simulink model "RADTRANS001"  (R2020b)
settings: Solver=VariableStepAuto  StartTime=0.0  StopTime=10.0  RelTol=1e-3
undefined symbols (not defined in the file): Line_110_C, Line_110_L, Line_110_R, Line_220_C, Line_220_L, Line_220_R, Line_35_C, Line_35_L, Line_35_R, Line_6_L, Line_6_R, Sys_f_Hz, Sys_V_net_kV, Tr_110_35_L_pu, Tr_110_35_R_pu, Tr_110_35_Sn_VA, Tr_110_35_V_HV_kV, Tr_110_35_V_LV_kV, Tr_110_6_L_pu, Tr_110_6_R_pu, Tr_110_6_Sn_VA, Tr_110_6_V_HV_kV, Tr_110_6_V_LV_kV, Tr_220_110_L_pu, Tr_220_110_R_pu, Tr_220_110_Sn_VA, Tr_220_110_V_HV_kV, Tr_220_110_V_LV_kV, Tr_35_04_L_pu, Tr_35_04_R_pu, Tr_35_04_Sn_VA, Tr_35_04_V_HV_kV, Tr_35_04_V_LV_kV, Tr_6_04_L_pu, Tr_6_04_R_pu, Tr_6_04_Sn_VA, Tr_6_04_V_HV_kV, Tr_6_04_V_LV_kV, Ts_powergui
libraries: dspstat3 x240, powerlib x169, powerlib_meascontrol x60
(part 4 of 6)

== system RADTRANS001/M_IN_Город_5_2 ==
  Iptg_55 : Display
      settings: Format=bank
  PQptg_55 : Scope  NumInputPorts=2
  "Power0 (3ph, Instantaneous)" : powerlib_meascontrol/Measurements/Power (3ph, Instantaneous)
  Pptg_55 : Display
      settings: Format=bank
  Qptg_55 : Display
      settings: Format=bank
  RMS3 : dspstat3/RMS  run=off  directionMode=Each column  dimension=1  InputProcessing=Columns as channels (frame based)  reset_popup=None
  RMS4 : dspstat3/RMS  run=off  directionMode=Each column  dimension=1  InputProcessing=Columns as channels (frame based)  reset_popup=None
  RMS55 : dspstat3/RMS  run=off  directionMode=Each column  dimension=1  InputProcessing=Columns as channels (frame based)  reset_popup=None
  RMSpt_55 : dspstat3/RMS  run=off  directionMode=Each column  dimension=1  InputProcessing=Columns as channels (frame based)  reset_popup=None
  Real-Ima to Complex : RealImagToComplex
  S : Abs
  SSptg_55 : Scope
  Sptg_55 : Display
      settings: Format=bank
  Three-Phase V-I Measurementpt_55 : powerlib/Measurements/Three-Phase V-I Measurement  VoltageMeasurement=phase-to-ground  SetLabelV=off  LabelV=Vabc  Vpu=off  VpuLL=off  CurrentMeasurement=yes  SetLabelI=off  LabelI=Iabc  Ipu=off  Pbase=100e6  Vbase=500e3  OutputType=Complex  PhasorSimulation=off  PSBequivalent=0
  UIptg_55 : Scope  NumInputPorts=2
  Uptg_55 : Display
      settings: Format=bank
  a : PMIOPort  Side=Right
  b : PMIOPort  Port=2  Side=Right
  c : PMIOPort  Port=3  Side=Right
  A : PMIOPort  Port=4  Side=Left
  B : PMIOPort  Port=5  Side=Left
  C : PMIOPort  Port=6  Side=Left
  tag scope: I_ptg_55=global, P_ptg_55=global, Q_ptg_55=global, S_ptg_55=global, U_ptg_55=global
  wires:
  S/1 -> [S_ptg_55]
  Real-Ima to Complex/1 -> S/1
  [S_ptg_55] -> Sptg_55/1
  [S_ptg_55] -> SSptg_55/1
  [P_ptg_55] -> RMSpt_55/1
  RMSpt_55/1 -> Pptg_55/1
  RMS55/1 -> Qptg_55/1
  [U_ptg_55] -> RMS3/1
  RMS3/1 -> Uptg_55/1
  [P_ptg_55] -> Real-Ima to Complex/1
  [Q_ptg_55] -> RMS55/1
  [I_ptg_55] -> RMS4/1
  RMS4/1 -> Iptg_55/1
  [U_ptg_55] -> UIptg_55/1  "U"
  [P_ptg_55] -> PQptg_55/1  "P"
  [I_ptg_55] -> UIptg_55/2  "I"
  Three-Phase V-I Measurementpt_55/1 -> [U_ptg_55]
  [Q_ptg_55] -> Real-Ima to Complex/2
  Three-Phase V-I Measurementpt_55/2 -> [I_ptg_55]
  [U_ptg_55] -> "Power0 (3ph, Instantaneous)"/1
  [I_ptg_55] -> "Power0 (3ph, Instantaneous)"/2
  "Power0 (3ph, Instantaneous)"/2 -> [Q_ptg_55]
  "Power0 (3ph, Instantaneous)"/1 -> [P_ptg_55]
  [Q_ptg_55] -> PQptg_55/2  "Q"
  connections:
  Three-Phase V-I Measurementpt_55/LConn1 -- A/RConn1
  Three-Phase V-I Measurementpt_55/RConn1 -- a/RConn1
  Three-Phase V-I Measurementpt_55/LConn2 -- B/RConn1
  Three-Phase V-I Measurementpt_55/LConn3 -- C/RConn1
  Three-Phase V-I Measurementpt_55/RConn3 -- c/RConn1
  Three-Phase V-I Measurementpt_55/RConn2 -- b/RConn1

== system RADTRANS001/M_IN_Город_5_3 ==
  Iptg_57 : Display
      settings: Format=bank
  PQptg_57 : Scope  NumInputPorts=2
  "Power0 (3ph, Instantaneous)" : powerlib_meascontrol/Measurements/Power (3ph, Instantaneous)
  Pptg_57 : Display
      settings: Format=bank
  Qptg_57 : Display
      settings: Format=bank
  RMS3 : dspstat3/RMS  run=off  directionMode=Each column  dimension=1  InputProcessing=Columns as channels (frame based)  reset_popup=None
  RMS4 : dspstat3/RMS  run=off  directionMode=Each column  dimension=1  InputProcessing=Columns as channels (frame based)  reset_popup=None
  RMS57 : dspstat3/RMS  run=off  directionMode=Each column  dimension=1  InputProcessing=Columns as channels (frame based)  reset_popup=None
  RMSpt_57 : dspstat3/RMS  run=off  directionMode=Each column  dimension=1  InputProcessing=Columns as channels (frame based)  reset_popup=None
  Real-Ima to Complex : RealImagToComplex
  S : Abs
  SSptg_57 : Scope
  Sptg_57 : Display
      settings: Format=bank
  Three-Phase V-I Measurementpt_57 : powerlib/Measurements/Three-Phase V-I Measurement  VoltageMeasurement=phase-to-ground  SetLabelV=off  LabelV=Vabc  Vpu=off  VpuLL=off  CurrentMeasurement=yes  SetLabelI=off  LabelI=Iabc  Ipu=off  Pbase=100e6  Vbase=500e3  OutputType=Complex  PhasorSimulation=off  PSBequivalent=0
  UIptg_57 : Scope  NumInputPorts=2
  Uptg_57 : Display
      settings: Format=bank
  a : PMIOPort  Side=Right
  b : PMIOPort  Port=2  Side=Right
  c : PMIOPort  Port=3  Side=Right
  A : PMIOPort  Port=4  Side=Left
  B : PMIOPort  Port=5  Side=Left
  C : PMIOPort  Port=6  Side=Left
  tag scope: I_ptg_57=global, P_ptg_57=global, Q_ptg_57=global, S_ptg_57=global, U_ptg_57=global
  wires:
  S/1 -> [S_ptg_57]
  Real-Ima to Complex/1 -> S/1
  [S_ptg_57] -> Sptg_57/1
  [S_ptg_57] -> SSptg_57/1
  [P_ptg_57] -> RMSpt_57/1
  RMSpt_57/1 -> Pptg_57/1
  RMS57/1 -> Qptg_57/1
  [U_ptg_57] -> RMS3/1
  RMS3/1 -> Uptg_57/1
  [P_ptg_57] -> Real-Ima to Complex/1
  [Q_ptg_57] -> RMS57/1
  [I_ptg_57] -> RMS4/1
  RMS4/1 -> Iptg_57/1
  [U_ptg_57] -> UIptg_57/1  "U"
  [P_ptg_57] -> PQptg_57/1  "P"
  [I_ptg_57] -> UIptg_57/2  "I"
  Three-Phase V-I Measurementpt_57/1 -> [U_ptg_57]
  [Q_ptg_57] -> Real-Ima to Complex/2
  Three-Phase V-I Measurementpt_57/2 -> [I_ptg_57]
  [U_ptg_57] -> "Power0 (3ph, Instantaneous)"/1
  [I_ptg_57] -> "Power0 (3ph, Instantaneous)"/2
  "Power0 (3ph, Instantaneous)"/2 -> [Q_ptg_57]
  "Power0 (3ph, Instantaneous)"/1 -> [P_ptg_57]
  [Q_ptg_57] -> PQptg_57/2  "Q"
  connections:
  Three-Phase V-I Measurementpt_57/LConn1 -- A/RConn1
  Three-Phase V-I Measurementpt_57/RConn1 -- a/RConn1
  Three-Phase V-I Measurementpt_57/LConn2 -- B/RConn1
  Three-Phase V-I Measurementpt_57/LConn3 -- C/RConn1
  Three-Phase V-I Measurementpt_57/RConn3 -- c/RConn1
  Three-Phase V-I Measurementpt_57/RConn2 -- b/RConn1

== system RADTRANS001/M_IN_Город_5_4 ==
  Iptg_59 : Display
      settings: Format=bank
  PQptg_59 : Scope  NumInputPorts=2
  "Power0 (3ph, Instantaneous)" : powerlib_meascontrol/Measurements/Power (3ph, Instantaneous)
  Pptg_59 : Display
      settings: Format=bank
  Qptg_59 : Display
      settings: Format=bank
  RMS3 : dspstat3/RMS  run=off  directionMode=Each column  dimension=1  InputProcessing=Columns as channels (frame based)  reset_popup=None
  RMS4 : dspstat3/RMS  run=off  directionMode=Each column  dimension=1  InputProcessing=Columns as channels (frame based)  reset_popup=None
  RMS59 : dspstat3/RMS  run=off  directionMode=Each column  dimension=1  InputProcessing=Columns as channels (frame based)  reset_popup=None
  RMSpt_59 : dspstat3/RMS  run=off  directionMode=Each column  dimension=1  InputProcessing=Columns as channels (frame based)  reset_popup=None
  Real-Ima to Complex : RealImagToComplex
  S : Abs
  SSptg_59 : Scope
  Sptg_59 : Display
      settings: Format=bank
  Three-Phase V-I Measurementpt_59 : powerlib/Measurements/Three-Phase V-I Measurement  VoltageMeasurement=phase-to-ground  SetLabelV=off  LabelV=Vabc  Vpu=off  VpuLL=off  CurrentMeasurement=yes  SetLabelI=off  LabelI=Iabc  Ipu=off  Pbase=100e6  Vbase=500e3  OutputType=Complex  PhasorSimulation=off  PSBequivalent=0
  UIptg_59 : Scope  NumInputPorts=2
  Uptg_59 : Display
      settings: Format=bank
  a : PMIOPort  Side=Right
  b : PMIOPort  Port=2  Side=Right
  c : PMIOPort  Port=3  Side=Right
  A : PMIOPort  Port=4  Side=Left
  B : PMIOPort  Port=5  Side=Left
  C : PMIOPort  Port=6  Side=Left
  tag scope: I_ptg_59=global, P_ptg_59=global, Q_ptg_59=global, S_ptg_59=global, U_ptg_59=global
  wires:
  S/1 -> [S_ptg_59]
  Real-Ima to Complex/1 -> S/1
  [S_ptg_59] -> Sptg_59/1
  [S_ptg_59] -> SSptg_59/1
  [P_ptg_59] -> RMSpt_59/1
  RMSpt_59/1 -> Pptg_59/1
  RMS59/1 -> Qptg_59/1
  [U_ptg_59] -> RMS3/1
  RMS3/1 -> Uptg_59/1
  [P_ptg_59] -> Real-Ima to Complex/1
  [Q_ptg_59] -> RMS59/1
  [I_ptg_59] -> RMS4/1
  RMS4/1 -> Iptg_59/1
  [U_ptg_59] -> UIptg_59/1  "U"
  [P_ptg_59] -> PQptg_59/1  "P"
  [I_ptg_59] -> UIptg_59/2  "I"
  Three-Phase V-I Measurementpt_59/1 -> [U_ptg_59]
  [Q_ptg_59] -> Real-Ima to Complex/2
  Three-Phase V-I Measurementpt_59/2 -> [I_ptg_59]
  [U_ptg_59] -> "Power0 (3ph, Instantaneous)"/1
  [I_ptg_59] -> "Power0 (3ph, Instantaneous)"/2
  "Power0 (3ph, Instantaneous)"/2 -> [Q_ptg_59]
  "Power0 (3ph, Instantaneous)"/1 -> [P_ptg_59]
  [Q_ptg_59] -> PQptg_59/2  "Q"
  connections:
  Three-Phase V-I Measurementpt_59/LConn1 -- A/RConn1
  Three-Phase V-I Measurementpt_59/RConn1 -- a/RConn1
  Three-Phase V-I Measurementpt_59/LConn2 -- B/RConn1
  Three-Phase V-I Measurementpt_59/LConn3 -- C/RConn1
  Three-Phase V-I Measurementpt_59/RConn3 -- c/RConn1
  Three-Phase V-I Measurementpt_59/RConn2 -- b/RConn1

== system RADTRANS001/M_IN_Завод_1_1 ==
  Iptg_1 : Display
      settings: Format=bank
  PQptg_1 : Scope  NumInputPorts=2
  "Power0 (3ph, Instantaneous)" : powerlib_meascontrol/Measurements/Power (3ph, Instantaneous)
  Pptg_1 : Display
      settings: Format=bank
  Qptg_1 : Display
      settings: Format=bank
  RMS1 : dspstat3/RMS  run=off  directionMode=Each column  dimension=1  InputProcessing=Columns as channels (frame based)  reset_popup=None
  RMS3 : dspstat3/RMS  run=off  directionMode=Each column  dimension=1  InputProcessing=Columns as channels (frame based)  reset_popup=None
  RMS4 : dspstat3/RMS  run=off  directionMode=Each column  dimension=1  InputProcessing=Columns as channels (frame based)  reset_popup=None
  RMSpt_1 : dspstat3/RMS  run=off  directionMode=Each column  dimension=1  InputProcessing=Columns as channels (frame based)  reset_popup=None
  Real-Ima to Complex : RealImagToComplex
  S : Abs
  SSptg_1 : Scope
  Sptg_1 : Display
      settings: Format=bank
  Three-Phase V-I Measurementpt_1 : powerlib/Measurements/Three-Phase V-I Measurement  VoltageMeasurement=phase-to-ground  SetLabelV=off  LabelV=Vabc  Vpu=off  VpuLL=off  CurrentMeasurement=yes  SetLabelI=off  LabelI=Iabc  Ipu=off  Pbase=100e6  Vbase=500e3  OutputType=Complex  PhasorSimulation=off  PSBequivalent=0
  UIptg_1 : Scope  NumInputPorts=2
  Uptg_1 : Display
      settings: Format=bank
  a : PMIOPort  Side=Right
  b : PMIOPort  Port=2  Side=Right
  c : PMIOPort  Port=3  Side=Right
  A : PMIOPort  Port=4  Side=Left
  B : PMIOPort  Port=5  Side=Left
  C : PMIOPort  Port=6  Side=Left
  tag scope: I_ptg_1=global, P_ptg_1=global, Q_ptg_1=global, S_ptg_1=global, U_ptg_1=global
  wires:
  S/1 -> [S_ptg_1]
  Real-Ima to Complex/1 -> S/1
  [S_ptg_1] -> Sptg_1/1
  [S_ptg_1] -> SSptg_1/1
  [P_ptg_1] -> RMSpt_1/1
  RMSpt_1/1 -> Pptg_1/1
  RMS1/1 -> Qptg_1/1
  [U_ptg_1] -> RMS3/1
  RMS3/1 -> Uptg_1/1
  [P_ptg_1] -> Real-Ima to Complex/1
  [Q_ptg_1] -> RMS1/1
  [I_ptg_1] -> RMS4/1
  RMS4/1 -> Iptg_1/1
  [U_ptg_1] -> UIptg_1/1  "U"
  [P_ptg_1] -> PQptg_1/1  "P"
  [I_ptg_1] -> UIptg_1/2  "I"
  Three-Phase V-I Measurementpt_1/1 -> [U_ptg_1]
  [Q_ptg_1] -> Real-Ima to Complex/2
  Three-Phase V-I Measurementpt_1/2 -> [I_ptg_1]
  [U_ptg_1] -> "Power0 (3ph, Instantaneous)"/1
  [I_ptg_1] -> "Power0 (3ph, Instantaneous)"/2
  "Power0 (3ph, Instantaneous)"/2 -> [Q_ptg_1]
  "Power0 (3ph, Instantaneous)"/1 -> [P_ptg_1]
  [Q_ptg_1] -> PQptg_1/2  "Q"
  connections:
  Three-Phase V-I Measurementpt_1/LConn1 -- A/RConn1
  Three-Phase V-I Measurementpt_1/RConn1 -- a/RConn1
  Three-Phase V-I Measurementpt_1/LConn2 -- B/RConn1
  Three-Phase V-I Measurementpt_1/LConn3 -- C/RConn1
  Three-Phase V-I Measurementpt_1/RConn3 -- c/RConn1
  Three-Phase V-I Measurementpt_1/RConn2 -- b/RConn1

== system RADTRANS001/M_IN_Завод_1_2 ==
  Iptg_3 : Display
      settings: Format=bank
  PQptg_3 : Scope  NumInputPorts=2
  "Power0 (3ph, Instantaneous)" : powerlib_meascontrol/Measurements/Power (3ph, Instantaneous)
  Pptg_3 : Display
      settings: Format=bank
  Qptg_3 : Display
      settings: Format=bank
  RMS0 : dspstat3/RMS  run=off  directionMode=Each column  dimension=1  InputProcessing=Columns as channels (frame based)  reset_popup=None
  RMS3 : dspstat3/RMS  run=off  directionMode=Each column  dimension=1  InputProcessing=Columns as channels (frame based)  reset_popup=None
  RMS4 : dspstat3/RMS  run=off  directionMode=Each column  dimension=1  InputProcessing=Columns as channels (frame based)  reset_popup=None
  RMSpt_3 : dspstat3/RMS  run=off  directionMode=Each column  dimension=1  InputProcessing=Columns as channels (frame based)  reset_popup=None
  Real-Ima to Complex : RealImagToComplex
  S : Abs
  SSptg_3 : Scope
  Sptg_3 : Display
      settings: Format=bank
  Three-Phase V-I Measurementpt_3 : powerlib/Measurements/Three-Phase V-I Measurement  VoltageMeasurement=phase-to-ground  SetLabelV=off  LabelV=Vabc  Vpu=off  VpuLL=off  CurrentMeasurement=yes  SetLabelI=off  LabelI=Iabc  Ipu=off  Pbase=100e6  Vbase=500e3  OutputType=Complex  PhasorSimulation=off  PSBequivalent=0
  UIptg_3 : Scope  NumInputPorts=2
  Uptg_3 : Display
      settings: Format=bank
  a : PMIOPort  Side=Right
  b : PMIOPort  Port=2  Side=Right
  c : PMIOPort  Port=3  Side=Right
  A : PMIOPort  Port=4  Side=Left
  B : PMIOPort  Port=5  Side=Left
  C : PMIOPort  Port=6  Side=Left
  tag scope: I_ptg_3=global, P_ptg_3=global, Q_ptg_3=global, S_ptg_3=global, U_ptg_3=global
  wires:
  S/1 -> [S_ptg_3]
  Real-Ima to Complex/1 -> S/1
  [S_ptg_3] -> Sptg_3/1
  [S_ptg_3] -> SSptg_3/1
  [P_ptg_3] -> RMSpt_3/1
  RMSpt_3/1 -> Pptg_3/1
  RMS0/1 -> Qptg_3/1
  [U_ptg_3] -> RMS3/1
  RMS3/1 -> Uptg_3/1
  [P_ptg_3] -> Real-Ima to Complex/1
  [Q_ptg_3] -> RMS0/1
  [I_ptg_3] -> RMS4/1
  RMS4/1 -> Iptg_3/1
  [U_ptg_3] -> UIptg_3/1  "U"
  [P_ptg_3] -> PQptg_3/1  "P"
  [I_ptg_3] -> UIptg_3/2  "I"
  Three-Phase V-I Measurementpt_3/1 -> [U_ptg_3]
  [Q_ptg_3] -> Real-Ima to Complex/2
  Three-Phase V-I Measurementpt_3/2 -> [I_ptg_3]
  [U_ptg_3] -> "Power0 (3ph, Instantaneous)"/1
  [I_ptg_3] -> "Power0 (3ph, Instantaneous)"/2
  "Power0 (3ph, Instantaneous)"/2 -> [Q_ptg_3]
  "Power0 (3ph, Instantaneous)"/1 -> [P_ptg_3]
  [Q_ptg_3] -> PQptg_3/2  "Q"
  connections:
  Three-Phase V-I Measurementpt_3/LConn1 -- A/RConn1
  Three-Phase V-I Measurementpt_3/RConn1 -- a/RConn1
  Three-Phase V-I Measurementpt_3/LConn2 -- B/RConn1
  Three-Phase V-I Measurementpt_3/LConn3 -- C/RConn1
  Three-Phase V-I Measurementpt_3/RConn3 -- c/RConn1
  Three-Phase V-I Measurementpt_3/RConn2 -- b/RConn1

== system RADTRANS001/M_IN_Завод_2_1 ==
  Iptg_13 : Display
      settings: Format=bank
  PQptg_13 : Scope  NumInputPorts=2
  "Power0 (3ph, Instantaneous)" : powerlib_meascontrol/Measurements/Power (3ph, Instantaneous)
  Pptg_13 : Display
      settings: Format=bank
  Qptg_13 : Display
      settings: Format=bank
  RMS13 : dspstat3/RMS  run=off  directionMode=Each column  dimension=1  InputProcessing=Columns as channels (frame based)  reset_popup=None
  RMS3 : dspstat3/RMS  run=off  directionMode=Each column  dimension=1  InputProcessing=Columns as channels (frame based)  reset_popup=None
  RMS4 : dspstat3/RMS  run=off  directionMode=Each column  dimension=1  InputProcessing=Columns as channels (frame based)  reset_popup=None
  RMSpt_13 : dspstat3/RMS  run=off  directionMode=Each column  dimension=1  InputProcessing=Columns as channels (frame based)  reset_popup=None
  Real-Ima to Complex : RealImagToComplex
  S : Abs
  SSptg_13 : Scope
  Sptg_13 : Display
      settings: Format=bank
  Three-Phase V-I Measurementpt_13 : powerlib/Measurements/Three-Phase V-I Measurement  VoltageMeasurement=phase-to-ground  SetLabelV=off  LabelV=Vabc  Vpu=off  VpuLL=off  CurrentMeasurement=yes  SetLabelI=off  LabelI=Iabc  Ipu=off  Pbase=100e6  Vbase=500e3  OutputType=Complex  PhasorSimulation=off  PSBequivalent=0
  UIptg_13 : Scope  NumInputPorts=2
  Uptg_13 : Display
      settings: Format=bank
  a : PMIOPort  Side=Right
  b : PMIOPort  Port=2  Side=Right
  c : PMIOPort  Port=3  Side=Right
  A : PMIOPort  Port=4  Side=Left
  B : PMIOPort  Port=5  Side=Left
  C : PMIOPort  Port=6  Side=Left
  tag scope: I_ptg_13=global, P_ptg_13=global, Q_ptg_13=global, S_ptg_13=global, U_ptg_13=global
  wires:
  S/1 -> [S_ptg_13]
  Real-Ima to Complex/1 -> S/1
  [S_ptg_13] -> Sptg_13/1
  [S_ptg_13] -> SSptg_13/1
  [P_ptg_13] -> RMSpt_13/1
  RMSpt_13/1 -> Pptg_13/1
  RMS13/1 -> Qptg_13/1
  [U_ptg_13] -> RMS3/1
  RMS3/1 -> Uptg_13/1
  [P_ptg_13] -> Real-Ima to Complex/1
  [Q_ptg_13] -> RMS13/1
  [I_ptg_13] -> RMS4/1
  RMS4/1 -> Iptg_13/1
  [U_ptg_13] -> UIptg_13/1  "U"
  [P_ptg_13] -> PQptg_13/1  "P"
  [I_ptg_13] -> UIptg_13/2  "I"
  Three-Phase V-I Measurementpt_13/1 -> [U_ptg_13]
  [Q_ptg_13] -> Real-Ima to Complex/2
  Three-Phase V-I Measurementpt_13/2 -> [I_ptg_13]
  [U_ptg_13] -> "Power0 (3ph, Instantaneous)"/1
  [I_ptg_13] -> "Power0 (3ph, Instantaneous)"/2
  "Power0 (3ph, Instantaneous)"/2 -> [Q_ptg_13]
  "Power0 (3ph, Instantaneous)"/1 -> [P_ptg_13]
  [Q_ptg_13] -> PQptg_13/2  "Q"
  connections:
  Three-Phase V-I Measurementpt_13/LConn1 -- A/RConn1
  Three-Phase V-I Measurementpt_13/RConn1 -- a/RConn1
  Three-Phase V-I Measurementpt_13/LConn2 -- B/RConn1
  Three-Phase V-I Measurementpt_13/LConn3 -- C/RConn1
  Three-Phase V-I Measurementpt_13/RConn3 -- c/RConn1
  Three-Phase V-I Measurementpt_13/RConn2 -- b/RConn1

== system RADTRANS001/M_IN_Завод_2_2 ==
  Iptg_15 : Display
      settings: Format=bank
  PQptg_15 : Scope  NumInputPorts=2
  "Power0 (3ph, Instantaneous)" : powerlib_meascontrol/Measurements/Power (3ph, Instantaneous)
  Pptg_15 : Display
      settings: Format=bank
  Qptg_15 : Display
      settings: Format=bank
  RMS15 : dspstat3/RMS  run=off  directionMode=Each column  dimension=1  InputProcessing=Columns as channels (frame based)  reset_popup=None
  RMS3 : dspstat3/RMS  run=off  directionMode=Each column  dimension=1  InputProcessing=Columns as channels (frame based)  reset_popup=None
  RMS4 : dspstat3/RMS  run=off  directionMode=Each column  dimension=1  InputProcessing=Columns as channels (frame based)  reset_popup=None
  RMSpt_15 : dspstat3/RMS  run=off  directionMode=Each column  dimension=1  InputProcessing=Columns as channels (frame based)  reset_popup=None
  Real-Ima to Complex : RealImagToComplex
  S : Abs
  SSptg_15 : Scope
  Sptg_15 : Display
      settings: Format=bank
  Three-Phase V-I Measurementpt_15 : powerlib/Measurements/Three-Phase V-I Measurement  VoltageMeasurement=phase-to-ground  SetLabelV=off  LabelV=Vabc  Vpu=off  VpuLL=off  CurrentMeasurement=yes  SetLabelI=off  LabelI=Iabc  Ipu=off  Pbase=100e6  Vbase=500e3  OutputType=Complex  PhasorSimulation=off  PSBequivalent=0
  UIptg_15 : Scope  NumInputPorts=2
  Uptg_15 : Display
      settings: Format=bank
  a : PMIOPort  Side=Right
  b : PMIOPort  Port=2  Side=Right
  c : PMIOPort  Port=3  Side=Right
  A : PMIOPort  Port=4  Side=Left
  B : PMIOPort  Port=5  Side=Left
  C : PMIOPort  Port=6  Side=Left
  tag scope: I_ptg_15=global, P_ptg_15=global, Q_ptg_15=global, S_ptg_15=global, U_ptg_15=global
  wires:
  S/1 -> [S_ptg_15]
  Real-Ima to Complex/1 -> S/1
  [S_ptg_15] -> Sptg_15/1
  [S_ptg_15] -> SSptg_15/1
  [P_ptg_15] -> RMSpt_15/1
  RMSpt_15/1 -> Pptg_15/1
  RMS15/1 -> Qptg_15/1
  [U_ptg_15] -> RMS3/1
  RMS3/1 -> Uptg_15/1
  [P_ptg_15] -> Real-Ima to Complex/1
  [Q_ptg_15] -> RMS15/1
  [I_ptg_15] -> RMS4/1
  RMS4/1 -> Iptg_15/1
  [U_ptg_15] -> UIptg_15/1  "U"
  [P_ptg_15] -> PQptg_15/1  "P"
  [I_ptg_15] -> UIptg_15/2  "I"
  Three-Phase V-I Measurementpt_15/1 -> [U_ptg_15]
  [Q_ptg_15] -> Real-Ima to Complex/2
  Three-Phase V-I Measurementpt_15/2 -> [I_ptg_15]
  [U_ptg_15] -> "Power0 (3ph, Instantaneous)"/1
  [I_ptg_15] -> "Power0 (3ph, Instantaneous)"/2
  "Power0 (3ph, Instantaneous)"/2 -> [Q_ptg_15]
  "Power0 (3ph, Instantaneous)"/1 -> [P_ptg_15]
  [Q_ptg_15] -> PQptg_15/2  "Q"
  connections:
  Three-Phase V-I Measurementpt_15/LConn1 -- A/RConn1
  Three-Phase V-I Measurementpt_15/RConn1 -- a/RConn1
  Three-Phase V-I Measurementpt_15/LConn2 -- B/RConn1
  Three-Phase V-I Measurementpt_15/LConn3 -- C/RConn1
  Three-Phase V-I Measurementpt_15/RConn3 -- c/RConn1
  Three-Phase V-I Measurementpt_15/RConn2 -- b/RConn1

== system RADTRANS001/M_IN_Завод_3_1 ==
  Iptg_25 : Display
      settings: Format=bank
  PQptg_25 : Scope  NumInputPorts=2
  "Power0 (3ph, Instantaneous)" : powerlib_meascontrol/Measurements/Power (3ph, Instantaneous)
  Pptg_25 : Display
      settings: Format=bank
  Qptg_25 : Display
      settings: Format=bank
  RMS25 : dspstat3/RMS  run=off  directionMode=Each column  dimension=1  InputProcessing=Columns as channels (frame based)  reset_popup=None
  RMS3 : dspstat3/RMS  run=off  directionMode=Each column  dimension=1  InputProcessing=Columns as channels (frame based)  reset_popup=None
  RMS4 : dspstat3/RMS  run=off  directionMode=Each column  dimension=1  InputProcessing=Columns as channels (frame based)  reset_popup=None
  RMSpt_25 : dspstat3/RMS  run=off  directionMode=Each column  dimension=1  InputProcessing=Columns as channels (frame based)  reset_popup=None
  Real-Ima to Complex : RealImagToComplex
  S : Abs
  SSptg_25 : Scope
  Sptg_25 : Display
      settings: Format=bank
  Three-Phase V-I Measurementpt_25 : powerlib/Measurements/Three-Phase V-I Measurement  VoltageMeasurement=phase-to-ground  SetLabelV=off  LabelV=Vabc  Vpu=off  VpuLL=off  CurrentMeasurement=yes  SetLabelI=off  LabelI=Iabc  Ipu=off  Pbase=100e6  Vbase=500e3  OutputType=Complex  PhasorSimulation=off  PSBequivalent=0
  UIptg_25 : Scope  NumInputPorts=2
  Uptg_25 : Display
      settings: Format=bank
  a : PMIOPort  Side=Right
  b : PMIOPort  Port=2  Side=Right
  c : PMIOPort  Port=3  Side=Right
  A : PMIOPort  Port=4  Side=Left
  B : PMIOPort  Port=5  Side=Left
  C : PMIOPort  Port=6  Side=Left
  tag scope: I_ptg_25=global, P_ptg_25=global, Q_ptg_25=global, S_ptg_25=global, U_ptg_25=global
  wires:
  S/1 -> [S_ptg_25]
  Real-Ima to Complex/1 -> S/1
  [S_ptg_25] -> Sptg_25/1
  [S_ptg_25] -> SSptg_25/1
  [P_ptg_25] -> RMSpt_25/1
  RMSpt_25/1 -> Pptg_25/1
  RMS25/1 -> Qptg_25/1
  [U_ptg_25] -> RMS3/1
  RMS3/1 -> Uptg_25/1
  [P_ptg_25] -> Real-Ima to Complex/1
  [Q_ptg_25] -> RMS25/1
  [I_ptg_25] -> RMS4/1
  RMS4/1 -> Iptg_25/1
  [U_ptg_25] -> UIptg_25/1  "U"
  [P_ptg_25] -> PQptg_25/1  "P"
  [I_ptg_25] -> UIptg_25/2  "I"
  Three-Phase V-I Measurementpt_25/1 -> [U_ptg_25]
  [Q_ptg_25] -> Real-Ima to Complex/2
  Three-Phase V-I Measurementpt_25/2 -> [I_ptg_25]
  [U_ptg_25] -> "Power0 (3ph, Instantaneous)"/1
  [I_ptg_25] -> "Power0 (3ph, Instantaneous)"/2
  "Power0 (3ph, Instantaneous)"/2 -> [Q_ptg_25]
  "Power0 (3ph, Instantaneous)"/1 -> [P_ptg_25]
  [Q_ptg_25] -> PQptg_25/2  "Q"
  connections:
  Three-Phase V-I Measurementpt_25/LConn1 -- A/RConn1
  Three-Phase V-I Measurementpt_25/RConn1 -- a/RConn1
  Three-Phase V-I Measurementpt_25/LConn2 -- B/RConn1
  Three-Phase V-I Measurementpt_25/LConn3 -- C/RConn1
  Three-Phase V-I Measurementpt_25/RConn3 -- c/RConn1
  Three-Phase V-I Measurementpt_25/RConn2 -- b/RConn1

== system RADTRANS001/M_IN_Завод_3_2 ==
  Iptg_27 : Display
      settings: Format=bank
  PQptg_27 : Scope  NumInputPorts=2
  "Power0 (3ph, Instantaneous)" : powerlib_meascontrol/Measurements/Power (3ph, Instantaneous)
  Pptg_27 : Display
      settings: Format=bank
  Qptg_27 : Display
      settings: Format=bank
  RMS27 : dspstat3/RMS  run=off  directionMode=Each column  dimension=1  InputProcessing=Columns as channels (frame based)  reset_popup=None
  RMS3 : dspstat3/RMS  run=off  directionMode=Each column  dimension=1  InputProcessing=Columns as channels (frame based)  reset_popup=None
  RMS4 : dspstat3/RMS  run=off  directionMode=Each column  dimension=1  InputProcessing=Columns as channels (frame based)  reset_popup=None
  RMSpt_27 : dspstat3/RMS  run=off  directionMode=Each column  dimension=1  InputProcessing=Columns as channels (frame based)  reset_popup=None
  Real-Ima to Complex : RealImagToComplex
  S : Abs
  SSptg_27 : Scope
  Sptg_27 : Display
      settings: Format=bank
  Three-Phase V-I Measurementpt_27 : powerlib/Measurements/Three-Phase V-I Measurement  VoltageMeasurement=phase-to-ground  SetLabelV=off  LabelV=Vabc  Vpu=off  VpuLL=off  CurrentMeasurement=yes  SetLabelI=off  LabelI=Iabc  Ipu=off  Pbase=100e6  Vbase=500e3  OutputType=Complex  PhasorSimulation=off  PSBequivalent=0
  UIptg_27 : Scope  NumInputPorts=2
  Uptg_27 : Display
      settings: Format=bank
  a : PMIOPort  Side=Right
  b : PMIOPort  Port=2  Side=Right
  c : PMIOPort  Port=3  Side=Right
  A : PMIOPort  Port=4  Side=Left
  B : PMIOPort  Port=5  Side=Left
  C : PMIOPort  Port=6  Side=Left
  tag scope: I_ptg_27=global, P_ptg_27=global, Q_ptg_27=global, S_ptg_27=global, U_ptg_27=global
  wires:
  S/1 -> [S_ptg_27]
  Real-Ima to Complex/1 -> S/1
  [S_ptg_27] -> Sptg_27/1
  [S_ptg_27] -> SSptg_27/1
  [P_ptg_27] -> RMSpt_27/1
  RMSpt_27/1 -> Pptg_27/1
  RMS27/1 -> Qptg_27/1
  [U_ptg_27] -> RMS3/1
  RMS3/1 -> Uptg_27/1
  [P_ptg_27] -> Real-Ima to Complex/1
  [Q_ptg_27] -> RMS27/1
  [I_ptg_27] -> RMS4/1
  RMS4/1 -> Iptg_27/1
  [U_ptg_27] -> UIptg_27/1  "U"
  [P_ptg_27] -> PQptg_27/1  "P"
  [I_ptg_27] -> UIptg_27/2  "I"
  Three-Phase V-I Measurementpt_27/1 -> [U_ptg_27]
  [Q_ptg_27] -> Real-Ima to Complex/2
  Three-Phase V-I Measurementpt_27/2 -> [I_ptg_27]
  [U_ptg_27] -> "Power0 (3ph, Instantaneous)"/1
  [I_ptg_27] -> "Power0 (3ph, Instantaneous)"/2
  "Power0 (3ph, Instantaneous)"/2 -> [Q_ptg_27]
  "Power0 (3ph, Instantaneous)"/1 -> [P_ptg_27]
  [Q_ptg_27] -> PQptg_27/2  "Q"
  connections:
  Three-Phase V-I Measurementpt_27/LConn1 -- A/RConn1
  Three-Phase V-I Measurementpt_27/RConn1 -- a/RConn1
  Three-Phase V-I Measurementpt_27/LConn2 -- B/RConn1
  Three-Phase V-I Measurementpt_27/LConn3 -- C/RConn1
  Three-Phase V-I Measurementpt_27/RConn3 -- c/RConn1
  Three-Phase V-I Measurementpt_27/RConn2 -- b/RConn1

== system RADTRANS001/M_IN_Завод_4_1 ==
  Iptg_37 : Display
      settings: Format=bank
  PQptg_37 : Scope  NumInputPorts=2
  "Power0 (3ph, Instantaneous)" : powerlib_meascontrol/Measurements/Power (3ph, Instantaneous)
  Pptg_37 : Display
      settings: Format=bank
  Qptg_37 : Display
      settings: Format=bank
  RMS3 : dspstat3/RMS  run=off  directionMode=Each column  dimension=1  InputProcessing=Columns as channels (frame based)  reset_popup=None
  RMS37 : dspstat3/RMS  run=off  directionMode=Each column  dimension=1  InputProcessing=Columns as channels (frame based)  reset_popup=None
  RMS4 : dspstat3/RMS  run=off  directionMode=Each column  dimension=1  InputProcessing=Columns as channels (frame based)  reset_popup=None
  RMSpt_37 : dspstat3/RMS  run=off  directionMode=Each column  dimension=1  InputProcessing=Columns as channels (frame based)  reset_popup=None
  Real-Ima to Complex : RealImagToComplex
  S : Abs
  SSptg_37 : Scope
  Sptg_37 : Display
      settings: Format=bank
  Three-Phase V-I Measurementpt_37 : powerlib/Measurements/Three-Phase V-I Measurement  VoltageMeasurement=phase-to-ground  SetLabelV=off  LabelV=Vabc  Vpu=off  VpuLL=off  CurrentMeasurement=yes  SetLabelI=off  LabelI=Iabc  Ipu=off  Pbase=100e6  Vbase=500e3  OutputType=Complex  PhasorSimulation=off  PSBequivalent=0
  UIptg_37 : Scope  NumInputPorts=2
  Uptg_37 : Display
      settings: Format=bank
  a : PMIOPort  Side=Right
  b : PMIOPort  Port=2  Side=Right
  c : PMIOPort  Port=3  Side=Right
  A : PMIOPort  Port=4  Side=Left
  B : PMIOPort  Port=5  Side=Left
  C : PMIOPort  Port=6  Side=Left
  tag scope: I_ptg_37=global, P_ptg_37=global, Q_ptg_37=global, S_ptg_37=global, U_ptg_37=global
  wires:
  S/1 -> [S_ptg_37]
  Real-Ima to Complex/1 -> S/1
  [S_ptg_37] -> Sptg_37/1
  [S_ptg_37] -> SSptg_37/1
  [P_ptg_37] -> RMSpt_37/1
  RMSpt_37/1 -> Pptg_37/1
  RMS37/1 -> Qptg_37/1
  [U_ptg_37] -> RMS3/1
  RMS3/1 -> Uptg_37/1
  [P_ptg_37] -> Real-Ima to Complex/1
  [Q_ptg_37] -> RMS37/1
  [I_ptg_37] -> RMS4/1
  RMS4/1 -> Iptg_37/1
  [U_ptg_37] -> UIptg_37/1  "U"
  [P_ptg_37] -> PQptg_37/1  "P"
  [I_ptg_37] -> UIptg_37/2  "I"
  Three-Phase V-I Measurementpt_37/1 -> [U_ptg_37]
  [Q_ptg_37] -> Real-Ima to Complex/2
  Three-Phase V-I Measurementpt_37/2 -> [I_ptg_37]
  [U_ptg_37] -> "Power0 (3ph, Instantaneous)"/1
  [I_ptg_37] -> "Power0 (3ph, Instantaneous)"/2
  "Power0 (3ph, Instantaneous)"/2 -> [Q_ptg_37]
  "Power0 (3ph, Instantaneous)"/1 -> [P_ptg_37]
  [Q_ptg_37] -> PQptg_37/2  "Q"
  connections:
  Three-Phase V-I Measurementpt_37/LConn1 -- A/RConn1
  Three-Phase V-I Measurementpt_37/RConn1 -- a/RConn1
  Three-Phase V-I Measurementpt_37/LConn2 -- B/RConn1
  Three-Phase V-I Measurementpt_37/LConn3 -- C/RConn1
  Three-Phase V-I Measurementpt_37/RConn3 -- c/RConn1
  Three-Phase V-I Measurementpt_37/RConn2 -- b/RConn1

== system RADTRANS001/M_IN_Завод_4_2 ==
  Iptg_39 : Display
      settings: Format=bank
  PQptg_39 : Scope  NumInputPorts=2
  "Power0 (3ph, Instantaneous)" : powerlib_meascontrol/Measurements/Power (3ph, Instantaneous)
  Pptg_39 : Display
      settings: Format=bank
  Qptg_39 : Display
      settings: Format=bank
  RMS3 : dspstat3/RMS  run=off  directionMode=Each column  dimension=1  InputProcessing=Columns as channels (frame based)  reset_popup=None
  RMS39 : dspstat3/RMS  run=off  directionMode=Each column  dimension=1  InputProcessing=Columns as channels (frame based)  reset_popup=None
  RMS4 : dspstat3/RMS  run=off  directionMode=Each column  dimension=1  InputProcessing=Columns as channels (frame based)  reset_popup=None
  RMSpt_39 : dspstat3/RMS  run=off  directionMode=Each column  dimension=1  InputProcessing=Columns as channels (frame based)  reset_popup=None
  Real-Ima to Complex : RealImagToComplex
  S : Abs
  SSptg_39 : Scope
  Sptg_39 : Display
      settings: Format=bank
  Three-Phase V-I Measurementpt_39 : powerlib/Measurements/Three-Phase V-I Measurement  VoltageMeasurement=phase-to-ground  SetLabelV=off  LabelV=Vabc  Vpu=off  VpuLL=off  CurrentMeasurement=yes  SetLabelI=off  LabelI=Iabc  Ipu=off  Pbase=100e6  Vbase=500e3  OutputType=Complex  PhasorSimulation=off  PSBequivalent=0
  UIptg_39 : Scope  NumInputPorts=2
  Uptg_39 : Display
      settings: Format=bank
  a : PMIOPort  Side=Right
  b : PMIOPort  Port=2  Side=Right
  c : PMIOPort  Port=3  Side=Right
  A : PMIOPort  Port=4  Side=Left
  B : PMIOPort  Port=5  Side=Left
  C : PMIOPort  Port=6  Side=Left
  tag scope: I_ptg_39=global, P_ptg_39=global, Q_ptg_39=global, S_ptg_39=global, U_ptg_39=global
  wires:
  S/1 -> [S_ptg_39]
  Real-Ima to Complex/1 -> S/1
  [S_ptg_39] -> Sptg_39/1
  [S_ptg_39] -> SSptg_39/1
  [P_ptg_39] -> RMSpt_39/1
  RMSpt_39/1 -> Pptg_39/1
  RMS39/1 -> Qptg_39/1
  [U_ptg_39] -> RMS3/1
  RMS3/1 -> Uptg_39/1
  [P_ptg_39] -> Real-Ima to Complex/1
  [Q_ptg_39] -> RMS39/1
  [I_ptg_39] -> RMS4/1
  RMS4/1 -> Iptg_39/1
  [U_ptg_39] -> UIptg_39/1  "U"
  [P_ptg_39] -> PQptg_39/1  "P"
  [I_ptg_39] -> UIptg_39/2  "I"
  Three-Phase V-I Measurementpt_39/1 -> [U_ptg_39]
  [Q_ptg_39] -> Real-Ima to Complex/2
  Three-Phase V-I Measurementpt_39/2 -> [I_ptg_39]
  [U_ptg_39] -> "Power0 (3ph, Instantaneous)"/1
  [I_ptg_39] -> "Power0 (3ph, Instantaneous)"/2
  "Power0 (3ph, Instantaneous)"/2 -> [Q_ptg_39]
  "Power0 (3ph, Instantaneous)"/1 -> [P_ptg_39]
  [Q_ptg_39] -> PQptg_39/2  "Q"
  connections:
  Three-Phase V-I Measurementpt_39/LConn1 -- A/RConn1
  Three-Phase V-I Measurementpt_39/RConn1 -- a/RConn1
  Three-Phase V-I Measurementpt_39/LConn2 -- B/RConn1
  Three-Phase V-I Measurementpt_39/LConn3 -- C/RConn1
  Three-Phase V-I Measurementpt_39/RConn3 -- c/RConn1
  Three-Phase V-I Measurementpt_39/RConn2 -- b/RConn1

== system RADTRANS001/M_IN_Завод_5_1 ==
  Iptg_49 : Display
      settings: Format=bank
  PQptg_49 : Scope  NumInputPorts=2
  "Power0 (3ph, Instantaneous)" : powerlib_meascontrol/Measurements/Power (3ph, Instantaneous)
  Pptg_49 : Display
      settings: Format=bank
  Qptg_49 : Display
      settings: Format=bank
  RMS3 : dspstat3/RMS  run=off  directionMode=Each column  dimension=1  InputProcessing=Columns as channels (frame based)  reset_popup=None
  RMS4 : dspstat3/RMS  run=off  directionMode=Each column  dimension=1  InputProcessing=Columns as channels (frame based)  reset_popup=None
  RMS49 : dspstat3/RMS  run=off  directionMode=Each column  dimension=1  InputProcessing=Columns as channels (frame based)  reset_popup=None
  RMSpt_49 : dspstat3/RMS  run=off  directionMode=Each column  dimension=1  InputProcessing=Columns as channels (frame based)  reset_popup=None
  Real-Ima to Complex : RealImagToComplex
  S : Abs
  SSptg_49 : Scope
  Sptg_49 : Display
      settings: Format=bank
  Three-Phase V-I Measurementpt_49 : powerlib/Measurements/Three-Phase V-I Measurement  VoltageMeasurement=phase-to-ground  SetLabelV=off  LabelV=Vabc  Vpu=off  VpuLL=off  CurrentMeasurement=yes  SetLabelI=off  LabelI=Iabc  Ipu=off  Pbase=100e6  Vbase=500e3  OutputType=Complex  PhasorSimulation=off  PSBequivalent=0
  UIptg_49 : Scope  NumInputPorts=2
  Uptg_49 : Display
      settings: Format=bank
  a : PMIOPort  Side=Right
  b : PMIOPort  Port=2  Side=Right
  c : PMIOPort  Port=3  Side=Right
  A : PMIOPort  Port=4  Side=Left
  B : PMIOPort  Port=5  Side=Left
  C : PMIOPort  Port=6  Side=Left
  tag scope: I_ptg_49=global, P_ptg_49=global, Q_ptg_49=global, S_ptg_49=global, U_ptg_49=global
  wires:
  S/1 -> [S_ptg_49]
  Real-Ima to Complex/1 -> S/1
  [S_ptg_49] -> Sptg_49/1
  [S_ptg_49] -> SSptg_49/1
  [P_ptg_49] -> RMSpt_49/1
  RMSpt_49/1 -> Pptg_49/1
  RMS49/1 -> Qptg_49/1
  [U_ptg_49] -> RMS3/1
  RMS3/1 -> Uptg_49/1
  [P_ptg_49] -> Real-Ima to Complex/1
  [Q_ptg_49] -> RMS49/1
  [I_ptg_49] -> RMS4/1
  RMS4/1 -> Iptg_49/1
  [U_ptg_49] -> UIptg_49/1  "U"
  [P_ptg_49] -> PQptg_49/1  "P"
  [I_ptg_49] -> UIptg_49/2  "I"
  Three-Phase V-I Measurementpt_49/1 -> [U_ptg_49]
  [Q_ptg_49] -> Real-Ima to Complex/2
  Three-Phase V-I Measurementpt_49/2 -> [I_ptg_49]
  [U_ptg_49] -> "Power0 (3ph, Instantaneous)"/1
  [I_ptg_49] -> "Power0 (3ph, Instantaneous)"/2
  "Power0 (3ph, Instantaneous)"/2 -> [Q_ptg_49]
  "Power0 (3ph, Instantaneous)"/1 -> [P_ptg_49]
  [Q_ptg_49] -> PQptg_49/2  "Q"
  connections:
  Three-Phase V-I Measurementpt_49/LConn1 -- A/RConn1
  Three-Phase V-I Measurementpt_49/RConn1 -- a/RConn1
  Three-Phase V-I Measurementpt_49/LConn2 -- B/RConn1
  Three-Phase V-I Measurementpt_49/LConn3 -- C/RConn1
  Three-Phase V-I Measurementpt_49/RConn3 -- c/RConn1
  Three-Phase V-I Measurementpt_49/RConn2 -- b/RConn1

== system RADTRANS001/M_IN_Завод_5_2 ==
  Iptg_51 : Display
      settings: Format=bank
  PQptg_51 : Scope  NumInputPorts=2
  "Power0 (3ph, Instantaneous)" : powerlib_meascontrol/Measurements/Power (3ph, Instantaneous)
  Pptg_51 : Display
      settings: Format=bank
  Qptg_51 : Display
      settings: Format=bank
  RMS3 : dspstat3/RMS  run=off  directionMode=Each column  dimension=1  InputProcessing=Columns as channels (frame based)  reset_popup=None
  RMS4 : dspstat3/RMS  run=off  directionMode=Each column  dimension=1  InputProcessing=Columns as channels (frame based)  reset_popup=None
  RMS51 : dspstat3/RMS  run=off  directionMode=Each column  dimension=1  InputProcessing=Columns as channels (frame based)  reset_popup=None
  RMSpt_51 : dspstat3/RMS  run=off  directionMode=Each column  dimension=1  InputProcessing=Columns as channels (frame based)  reset_popup=None
  Real-Ima to Complex : RealImagToComplex
  S : Abs
  SSptg_51 : Scope
  Sptg_51 : Display
      settings: Format=bank
  Three-Phase V-I Measurementpt_51 : powerlib/Measurements/Three-Phase V-I Measurement  VoltageMeasurement=phase-to-ground  SetLabelV=off  LabelV=Vabc  Vpu=off  VpuLL=off  CurrentMeasurement=yes  SetLabelI=off  LabelI=Iabc  Ipu=off  Pbase=100e6  Vbase=500e3  OutputType=Complex  PhasorSimulation=off  PSBequivalent=0
  UIptg_51 : Scope  NumInputPorts=2
  Uptg_51 : Display
      settings: Format=bank
  a : PMIOPort  Side=Right
  b : PMIOPort  Port=2  Side=Right
  c : PMIOPort  Port=3  Side=Right
  A : PMIOPort  Port=4  Side=Left
  B : PMIOPort  Port=5  Side=Left
  C : PMIOPort  Port=6  Side=Left
  tag scope: I_ptg_51=global, P_ptg_51=global, Q_ptg_51=global, S_ptg_51=global, U_ptg_51=global
  wires:
  S/1 -> [S_ptg_51]
  Real-Ima to Complex/1 -> S/1
  [S_ptg_51] -> Sptg_51/1
  [S_ptg_51] -> SSptg_51/1
  [P_ptg_51] -> RMSpt_51/1
  RMSpt_51/1 -> Pptg_51/1
  RMS51/1 -> Qptg_51/1
  [U_ptg_51] -> RMS3/1
  RMS3/1 -> Uptg_51/1
  [P_ptg_51] -> Real-Ima to Complex/1
  [Q_ptg_51] -> RMS51/1
  [I_ptg_51] -> RMS4/1
  RMS4/1 -> Iptg_51/1
  [U_ptg_51] -> UIptg_51/1  "U"
  [P_ptg_51] -> PQptg_51/1  "P"
  [I_ptg_51] -> UIptg_51/2  "I"
  Three-Phase V-I Measurementpt_51/1 -> [U_ptg_51]
  [Q_ptg_51] -> Real-Ima to Complex/2
  Three-Phase V-I Measurementpt_51/2 -> [I_ptg_51]
  [U_ptg_51] -> "Power0 (3ph, Instantaneous)"/1
  [I_ptg_51] -> "Power0 (3ph, Instantaneous)"/2
  "Power0 (3ph, Instantaneous)"/2 -> [Q_ptg_51]
  "Power0 (3ph, Instantaneous)"/1 -> [P_ptg_51]
  [Q_ptg_51] -> PQptg_51/2  "Q"
  connections:
  Three-Phase V-I Measurementpt_51/LConn1 -- A/RConn1
  Three-Phase V-I Measurementpt_51/RConn1 -- a/RConn1
  Three-Phase V-I Measurementpt_51/LConn2 -- B/RConn1
  Three-Phase V-I Measurementpt_51/LConn3 -- C/RConn1
  Three-Phase V-I Measurementpt_51/RConn3 -- c/RConn1
  Three-Phase V-I Measurementpt_51/RConn2 -- b/RConn1

== system RADTRANS001/M_OUT_Город_1_1 ==
  Iptg_6 : Display
      settings: Format=bank
  PQptg_6 : Scope  NumInputPorts=2
  "Power0 (3ph, Instantaneous)" : powerlib_meascontrol/Measurements/Power (3ph, Instantaneous)
  Pptg_6 : Display
      settings: Format=bank
  Qptg_6 : Display
      settings: Format=bank
  RMS3 : dspstat3/RMS  run=off  directionMode=Each column  dimension=1  InputProcessing=Columns as channels (frame based)  reset_popup=None
  RMS4 : dspstat3/RMS  run=off  directionMode=Each column  dimension=1  InputProcessing=Columns as channels (frame based)  reset_popup=None
  RMS6 : dspstat3/RMS  run=off  directionMode=Each column  dimension=1  InputProcessing=Columns as channels (frame based)  reset_popup=None
  RMSpt_6 : dspstat3/RMS  run=off  directionMode=Each column  dimension=1  InputProcessing=Columns as channels (frame based)  reset_popup=None
  Real-Ima to Complex : RealImagToComplex
  S : Abs
  SSptg_6 : Scope
  Sptg_6 : Display
      settings: Format=bank
  Three-Phase V-I Measurementpt_6 : powerlib/Measurements/Three-Phase V-I Measurement  VoltageMeasurement=phase-to-ground  SetLabelV=off  LabelV=Vabc  Vpu=off  VpuLL=off  CurrentMeasurement=yes  SetLabelI=off  LabelI=Iabc  Ipu=off  Pbase=100e6  Vbase=500e3  OutputType=Complex  PhasorSimulation=off  PSBequivalent=0
  UIptg_6 : Scope  NumInputPorts=2
  Uptg_6 : Display
      settings: Format=bank
  a : PMIOPort  Side=Right
  b : PMIOPort  Port=2  Side=Right
  c : PMIOPort  Port=3  Side=Right
  A : PMIOPort  Port=4  Side=Left
  B : PMIOPort  Port=5  Side=Left
  C : PMIOPort  Port=6  Side=Left
  tag scope: I_ptg_6=global, P_ptg_6=global, Q_ptg_6=global, S_ptg_6=global, U_ptg_6=global
  wires:
  S/1 -> [S_ptg_6]
  Real-Ima to Complex/1 -> S/1
  [S_ptg_6] -> Sptg_6/1
  [S_ptg_6] -> SSptg_6/1
  [P_ptg_6] -> RMSpt_6/1
  RMSpt_6/1 -> Pptg_6/1
  RMS6/1 -> Qptg_6/1
  [U_ptg_6] -> RMS3/1
  RMS3/1 -> Uptg_6/1
  [P_ptg_6] -> Real-Ima to Complex/1
  [Q_ptg_6] -> RMS6/1
  [I_ptg_6] -> RMS4/1
  RMS4/1 -> Iptg_6/1
  [U_ptg_6] -> UIptg_6/1  "U"
  [P_ptg_6] -> PQptg_6/1  "P"
  [I_ptg_6] -> UIptg_6/2  "I"
  Three-Phase V-I Measurementpt_6/1 -> [U_ptg_6]
  [Q_ptg_6] -> Real-Ima to Complex/2
  Three-Phase V-I Measurementpt_6/2 -> [I_ptg_6]
  [U_ptg_6] -> "Power0 (3ph, Instantaneous)"/1
  [I_ptg_6] -> "Power0 (3ph, Instantaneous)"/2
  "Power0 (3ph, Instantaneous)"/2 -> [Q_ptg_6]
  "Power0 (3ph, Instantaneous)"/1 -> [P_ptg_6]
  [Q_ptg_6] -> PQptg_6/2  "Q"
  connections:
  Three-Phase V-I Measurementpt_6/LConn1 -- A/RConn1
  Three-Phase V-I Measurementpt_6/RConn1 -- a/RConn1
  Three-Phase V-I Measurementpt_6/LConn2 -- B/RConn1
  Three-Phase V-I Measurementpt_6/LConn3 -- C/RConn1
  Three-Phase V-I Measurementpt_6/RConn3 -- c/RConn1
  Three-Phase V-I Measurementpt_6/RConn2 -- b/RConn1

== system RADTRANS001/M_OUT_Город_1_2 ==
  Iptg_8 : Display
      settings: Format=bank
  PQptg_8 : Scope  NumInputPorts=2
  "Power0 (3ph, Instantaneous)" : powerlib_meascontrol/Measurements/Power (3ph, Instantaneous)
  Pptg_8 : Display
      settings: Format=bank
  Qptg_8 : Display
      settings: Format=bank
  RMS3 : dspstat3/RMS  run=off  directionMode=Each column  dimension=1  InputProcessing=Columns as channels (frame based)  reset_popup=None
  RMS4 : dspstat3/RMS  run=off  directionMode=Each column  dimension=1  InputProcessing=Columns as channels (frame based)  reset_popup=None
  RMS8 : dspstat3/RMS  run=off  directionMode=Each column  dimension=1  InputProcessing=Columns as channels (frame based)  reset_popup=None
  RMSpt_8 : dspstat3/RMS  run=off  directionMode=Each column  dimension=1  InputProcessing=Columns as channels (frame based)  reset_popup=None
  Real-Ima to Complex : RealImagToComplex
  S : Abs
  SSptg_8 : Scope
  Sptg_8 : Display
      settings: Format=bank
  Three-Phase V-I Measurementpt_8 : powerlib/Measurements/Three-Phase V-I Measurement  VoltageMeasurement=phase-to-ground  SetLabelV=off  LabelV=Vabc  Vpu=off  VpuLL=off  CurrentMeasurement=yes  SetLabelI=off  LabelI=Iabc  Ipu=off  Pbase=100e6  Vbase=500e3  OutputType=Complex  PhasorSimulation=off  PSBequivalent=0
  UIptg_8 : Scope  NumInputPorts=2
  Uptg_8 : Display
      settings: Format=bank
  a : PMIOPort  Side=Right
  b : PMIOPort  Port=2  Side=Right
  c : PMIOPort  Port=3  Side=Right
  A : PMIOPort  Port=4  Side=Left
  B : PMIOPort  Port=5  Side=Left
  C : PMIOPort  Port=6  Side=Left
  tag scope: I_ptg_8=global, P_ptg_8=global, Q_ptg_8=global, S_ptg_8=global, U_ptg_8=global
  wires:
  S/1 -> [S_ptg_8]
  Real-Ima to Complex/1 -> S/1
  [S_ptg_8] -> Sptg_8/1
  [S_ptg_8] -> SSptg_8/1
  [P_ptg_8] -> RMSpt_8/1
  RMSpt_8/1 -> Pptg_8/1
  RMS8/1 -> Qptg_8/1
  [U_ptg_8] -> RMS3/1
  RMS3/1 -> Uptg_8/1
  [P_ptg_8] -> Real-Ima to Complex/1
  [Q_ptg_8] -> RMS8/1
  [I_ptg_8] -> RMS4/1
  RMS4/1 -> Iptg_8/1
  [U_ptg_8] -> UIptg_8/1  "U"
  [P_ptg_8] -> PQptg_8/1  "P"
  [I_ptg_8] -> UIptg_8/2  "I"
  Three-Phase V-I Measurementpt_8/1 -> [U_ptg_8]
  [Q_ptg_8] -> Real-Ima to Complex/2
  Three-Phase V-I Measurementpt_8/2 -> [I_ptg_8]
  [U_ptg_8] -> "Power0 (3ph, Instantaneous)"/1
  [I_ptg_8] -> "Power0 (3ph, Instantaneous)"/2
  "Power0 (3ph, Instantaneous)"/2 -> [Q_ptg_8]
  "Power0 (3ph, Instantaneous)"/1 -> [P_ptg_8]
  [Q_ptg_8] -> PQptg_8/2  "Q"
  connections:
  Three-Phase V-I Measurementpt_8/LConn1 -- A/RConn1
  Three-Phase V-I Measurementpt_8/RConn1 -- a/RConn1
  Three-Phase V-I Measurementpt_8/LConn2 -- B/RConn1
  Three-Phase V-I Measurementpt_8/LConn3 -- C/RConn1
  Three-Phase V-I Measurementpt_8/RConn3 -- c/RConn1
  Three-Phase V-I Measurementpt_8/RConn2 -- b/RConn1

== system RADTRANS001/M_OUT_Город_1_3 ==
  Iptg_10 : Display
      settings: Format=bank
  PQptg_10 : Scope  NumInputPorts=2
  "Power0 (3ph, Instantaneous)" : powerlib_meascontrol/Measurements/Power (3ph, Instantaneous)
  Pptg_10 : Display
      settings: Format=bank
  Qptg_10 : Display
      settings: Format=bank
  RMS10 : dspstat3/RMS  run=off  directionMode=Each column  dimension=1  InputProcessing=Columns as channels (frame based)  reset_popup=None
  RMS3 : dspstat3/RMS  run=off  directionMode=Each column  dimension=1  InputProcessing=Columns as channels (frame based)  reset_popup=None
  RMS4 : dspstat3/RMS  run=off  directionMode=Each column  dimension=1  InputProcessing=Columns as channels (frame based)  reset_popup=None
  RMSpt_10 : dspstat3/RMS  run=off  directionMode=Each column  dimension=1  InputProcessing=Columns as channels (frame based)  reset_popup=None
  Real-Ima to Complex : RealImagToComplex
  S : Abs
  SSptg_10 : Scope
  Sptg_10 : Display
      settings: Format=bank
  Three-Phase V-I Measurementpt_10 : powerlib/Measurements/Three-Phase V-I Measurement  VoltageMeasurement=phase-to-ground  SetLabelV=off  LabelV=Vabc  Vpu=off  VpuLL=off  CurrentMeasurement=yes  SetLabelI=off  LabelI=Iabc  Ipu=off  Pbase=100e6  Vbase=500e3  OutputType=Complex  PhasorSimulation=off  PSBequivalent=0
  UIptg_10 : Scope  NumInputPorts=2
  Uptg_10 : Display
      settings: Format=bank
  a : PMIOPort  Side=Right
  b : PMIOPort  Port=2  Side=Right
  c : PMIOPort  Port=3  Side=Right
  A : PMIOPort  Port=4  Side=Left
  B : PMIOPort  Port=5  Side=Left
  C : PMIOPort  Port=6  Side=Left
  tag scope: I_ptg_10=global, P_ptg_10=global, Q_ptg_10=global, S_ptg_10=global, U_ptg_10=global
  wires:
  S/1 -> [S_ptg_10]
  Real-Ima to Complex/1 -> S/1
  [S_ptg_10] -> Sptg_10/1
  [S_ptg_10] -> SSptg_10/1
  [P_ptg_10] -> RMSpt_10/1
  RMSpt_10/1 -> Pptg_10/1
  RMS10/1 -> Qptg_10/1
  [U_ptg_10] -> RMS3/1
  RMS3/1 -> Uptg_10/1
  [P_ptg_10] -> Real-Ima to Complex/1
  [Q_ptg_10] -> RMS10/1
  [I_ptg_10] -> RMS4/1
  RMS4/1 -> Iptg_10/1
  [U_ptg_10] -> UIptg_10/1  "U"
  [P_ptg_10] -> PQptg_10/1  "P"
  [I_ptg_10] -> UIptg_10/2  "I"
  Three-Phase V-I Measurementpt_10/1 -> [U_ptg_10]
  [Q_ptg_10] -> Real-Ima to Complex/2
  Three-Phase V-I Measurementpt_10/2 -> [I_ptg_10]
  [U_ptg_10] -> "Power0 (3ph, Instantaneous)"/1
  [I_ptg_10] -> "Power0 (3ph, Instantaneous)"/2
  "Power0 (3ph, Instantaneous)"/2 -> [Q_ptg_10]
  "Power0 (3ph, Instantaneous)"/1 -> [P_ptg_10]
  [Q_ptg_10] -> PQptg_10/2  "Q"
  connections:
  Three-Phase V-I Measurementpt_10/LConn1 -- A/RConn1
  Three-Phase V-I Measurementpt_10/RConn1 -- a/RConn1
  Three-Phase V-I Measurementpt_10/LConn2 -- B/RConn1
  Three-Phase V-I Measurementpt_10/LConn3 -- C/RConn1
  Three-Phase V-I Measurementpt_10/RConn3 -- c/RConn1
  Three-Phase V-I Measurementpt_10/RConn2 -- b/RConn1

== system RADTRANS001/M_OUT_Город_1_4 ==
  Iptg_12 : Display
      settings: Format=bank
  PQptg_12 : Scope  NumInputPorts=2
  "Power0 (3ph, Instantaneous)" : powerlib_meascontrol/Measurements/Power (3ph, Instantaneous)
  Pptg_12 : Display
      settings: Format=bank
  Qptg_12 : Display
      settings: Format=bank
  RMS12 : dspstat3/RMS  run=off  directionMode=Each column  dimension=1  InputProcessing=Columns as channels (frame based)  reset_popup=None
  RMS3 : dspstat3/RMS  run=off  directionMode=Each column  dimension=1  InputProcessing=Columns as channels (frame based)  reset_popup=None
  RMS4 : dspstat3/RMS  run=off  directionMode=Each column  dimension=1  InputProcessing=Columns as channels (frame based)  reset_popup=None
  RMSpt_12 : dspstat3/RMS  run=off  directionMode=Each column  dimension=1  InputProcessing=Columns as channels (frame based)  reset_popup=None
  Real-Ima to Complex : RealImagToComplex
  S : Abs
  SSptg_12 : Scope
  Sptg_12 : Display
      settings: Format=bank
  Three-Phase V-I Measurementpt_12 : powerlib/Measurements/Three-Phase V-I Measurement  VoltageMeasurement=phase-to-ground  SetLabelV=off  LabelV=Vabc  Vpu=off  VpuLL=off  CurrentMeasurement=yes  SetLabelI=off  LabelI=Iabc  Ipu=off  Pbase=100e6  Vbase=500e3  OutputType=Complex  PhasorSimulation=off  PSBequivalent=0
  UIptg_12 : Scope  NumInputPorts=2
  Uptg_12 : Display
      settings: Format=bank
  a : PMIOPort  Side=Right
  b : PMIOPort  Port=2  Side=Right
  c : PMIOPort  Port=3  Side=Right
  A : PMIOPort  Port=4  Side=Left
  B : PMIOPort  Port=5  Side=Left
  C : PMIOPort  Port=6  Side=Left
  tag scope: I_ptg_12=global, P_ptg_12=global, Q_ptg_12=global, S_ptg_12=global, U_ptg_12=global
  wires:
  S/1 -> [S_ptg_12]
  Real-Ima to Complex/1 -> S/1
  [S_ptg_12] -> Sptg_12/1
  [S_ptg_12] -> SSptg_12/1
  [P_ptg_12] -> RMSpt_12/1
  RMSpt_12/1 -> Pptg_12/1
  RMS12/1 -> Qptg_12/1
  [U_ptg_12] -> RMS3/1
  RMS3/1 -> Uptg_12/1
  [P_ptg_12] -> Real-Ima to Complex/1
  [Q_ptg_12] -> RMS12/1
  [I_ptg_12] -> RMS4/1
  RMS4/1 -> Iptg_12/1
  [U_ptg_12] -> UIptg_12/1  "U"
  [P_ptg_12] -> PQptg_12/1  "P"
  [I_ptg_12] -> UIptg_12/2  "I"
  Three-Phase V-I Measurementpt_12/1 -> [U_ptg_12]
  [Q_ptg_12] -> Real-Ima to Complex/2
  Three-Phase V-I Measurementpt_12/2 -> [I_ptg_12]
  [U_ptg_12] -> "Power0 (3ph, Instantaneous)"/1
  [I_ptg_12] -> "Power0 (3ph, Instantaneous)"/2
  "Power0 (3ph, Instantaneous)"/2 -> [Q_ptg_12]
  "Power0 (3ph, Instantaneous)"/1 -> [P_ptg_12]
  [Q_ptg_12] -> PQptg_12/2  "Q"
  connections:
  Three-Phase V-I Measurementpt_12/LConn1 -- A/RConn1
  Three-Phase V-I Measurementpt_12/RConn1 -- a/RConn1
  Three-Phase V-I Measurementpt_12/LConn2 -- B/RConn1
  Three-Phase V-I Measurementpt_12/LConn3 -- C/RConn1
  Three-Phase V-I Measurementpt_12/RConn3 -- c/RConn1
  Three-Phase V-I Measurementpt_12/RConn2 -- b/RConn1
